simulink model "SetButton"  (R2017a)
settings: Solver=VariableStepAuto  StartTime=0.0  StopTime=60  RelTol=1e-3
libraries: arduino_io_lib x4, simulink x3, dspstat3 x1
settings Model: Creator=enes_  LastModifiedBy=enes_

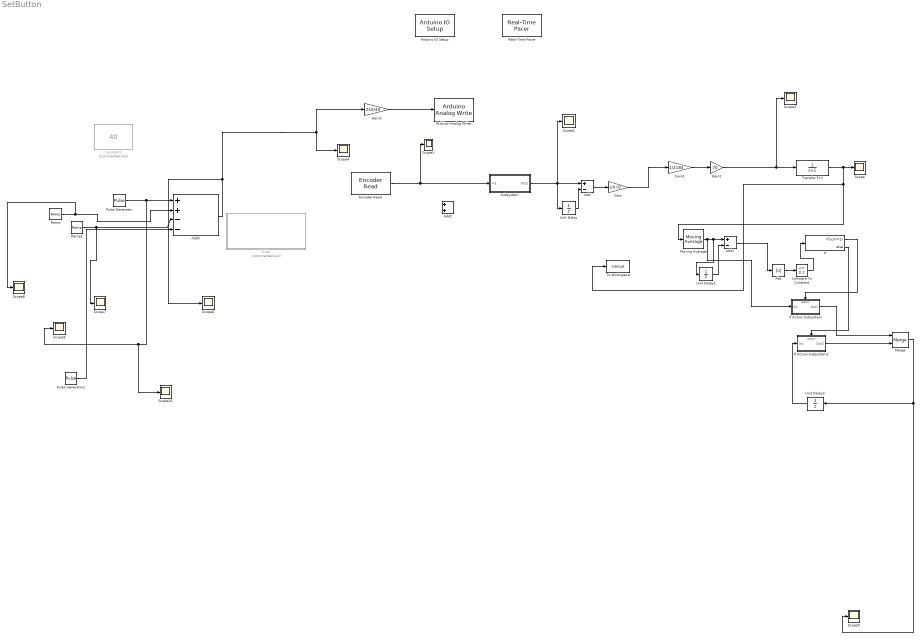
== system SetButton ==
  Abs : Abs
  Add : Sum  Inputs=+-
  Add1 : Sum  Inputs=+-
  Add2 : Sum
  Add3 : Sum  Inputs=++--
  Arduino Analog Write : arduino_io_lib/Arduino Analog Write  arduinoVar=Temporary arduino variable: Arduino1  arduinoPin=5  T=0.2
  Arduino IO Setup : arduino_io_lib/Arduino IO Setup  Priority=3  arduinoVar=Temporary arduino variable: Arduino1  workspaceVarName=a  comPort=COM4
  Compare To Constant : simulink/Logic and Bit Operations/Compare To Constant  relop=<=  const=0.2  OutDataTypeStr=boolean
  Constant1 : Constant  Commented=on  Value=40  SampleTime=0.02
  Encoder Read : arduino_io_lib/Encoder Read  arduinoVar=Temporary arduino variable: Arduino1  encNum=1  pinA=2  pinB=3  DbDl=1  T=0.02
  Gain : Gain  Gain=1/0.02
  Gain1 : Gain  Gain=1/2184
  Gain2 : Gain  Gain=70
  Gain3 : Gain  Gain=255/40
  If : If  IfExpression=u1==1
  If Action Subsystem : Subsystem  TreatAsAtomicUnit=on
  If Action Subsystem1 : Subsystem  TreatAsAtomicUnit=on
  Merge : Merge
  Moving Average : dspstat3/Moving Average  Method=Sliding window  SpecifyWindowLength=on  WindowLength=40  ForgettingFactor=0.9  SimulateUsing=Code generation
  Pulse Generator : DiscretePulseGenerator  Amplitude=0  Period=10  PulseWidth=10  PhaseDelay=40
  Pulse Generator1 : DiscretePulseGenerator  Amplitude=-40  Period=10  PulseWidth=10
  Ramp : simulink/Sources/Ramp  slope=1  start=0  X0=0
  Ramp1 : simulink/Sources/Ramp  slope=1  start=40  X0=40
  Real-Time Pacer : arduino_io_lib/Real-Time Pacer  simTimePerRealTime=1
  Scope{,1..10} (11 alike) : Scope
  Slider : Subsystem  Commented=on  DialogController=hmiCreateDDGDialog  IsWebBlock=on  mask(MWDashboardBlock){webBlockId=d8bc7804-6bab-4972-ab32-33c45766c117, webBlockType=slider, ShowInLibBrowser=on, ShowInitialText=on, HMISrcModelName=SetButton}
      mask prompts: webBlockId "WebBlock Id"; webBlockType "WebBlock Type"; HMISrcModelName "Source Model"
      mask help: SimulinkHMI:dialogs:SliderDialogDesc
      mask Help: helpview([docroot '/mapfiles/simulink.map'], 'hmi_slider')
      mask Display:
      | if strcmp(get_param(bdroot(gcb),'BlockDiagramType'), 'library')
      |     image([(matlabroot) '/toolbox/simulink/hmi/icons/Slider.png']);
      | end
  Subsystem : Subsystem
  To Workspace : ToWorkspace  VariableName=simout  SaveFormat=Timeseries  SampleTime=-1
  Transfer Fcn : TransferFcn  Denominator=[1 1]
  Unit Delay : UnitDelay  SampleTime=-1
  Unit Delay1 : UnitDelay  SampleTime=-1
  Unit Delay2 : UnitDelay  SampleTime=-1
  wires:
  Unit Delay/1 -> Add/2
  Add/1 -> Gain/1
  Gain/1 -> Gain1/1
  Gain1/1 -> Gain2/1
  Subsystem/1(Out1) -> Unit Delay/1, Scope2/1, Add/1
  Gain2/1 -> Transfer Fcn/1, Scope3/1
  Gain3/1 -> Arduino Analog Write/1
  Moving Average/1 -> If Action Subsystem/1(In1), Unit Delay1/1, Add1/1
  Unit Delay1/1 -> Add1/2
  Add1/1 -> Abs/1
  Abs/1 -> Compare To Constant/1
  Compare To Constant/1 -> If/1
  If/1 -> If Action Subsystem/Action
  If/2 -> If Action Subsystem1/Action
  If Action Subsystem/1(Out1) -> Merge/1
  Add3/1 -> Scope6/1, Scope4/1, Gain3/1
  If Action Subsystem1/1(Out1) -> Merge/2
  Merge/1 -> Unit Delay2/1, Scope5/1
  Transfer Fcn/1 -> To Workspace/1, Moving Average/1, Scope/1
  Encoder Read/1 -> Subsystem/1(In1), Scope1/1
  Pulse Generator/1 -> Scope10/1, Scope9/1, Add3/1
  Ramp/1 -> Scope8/1, Add3/2
  Ramp1/1 -> Scope7/1, Add3/3
  Pulse Generator1/1 -> Add3/4
  Unit Delay2/1 -> If Action Subsystem1/1(In1)

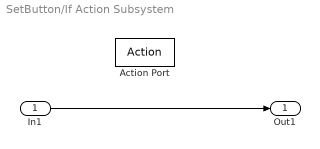
== system SetButton/If Action Subsystem ==
  In1 : Inport
  Action Port : ActionPort  ActionType=then
  Out1 : Outport
  wires:
  In1/1 -> Out1/1

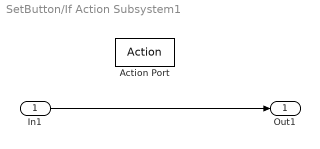
== system SetButton/If Action Subsystem1 ==
  In1 : Inport
  Action Port : ActionPort  ActionType=else
  Out1 : Outport
  wires:
  In1/1 -> Out1/1

== system SetButton/Slider ==

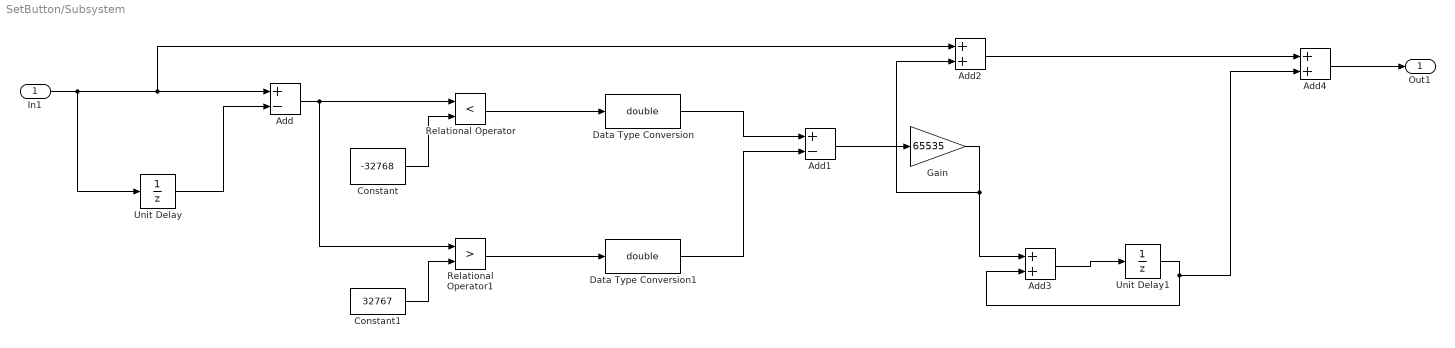
== system SetButton/Subsystem ==
  In1 : Inport
  Add : Sum  Inputs=+-
  Add1 : Sum  Inputs=+-
  Add2 : Sum
  Add3 : Sum
  Add4 : Sum
  Constant : Constant  Value=-32768
  Constant1 : Constant  Value=32767
  Data Type Conversion : DataTypeConversion  OutDataTypeStr=double
  Data Type Conversion1 : DataTypeConversion  OutDataTypeStr=double
  Gain : Gain  Gain=65535
  Relational Operator : RelationalOperator  Operator=<  OutDataTypeStr=boolean  RndMeth=Simplest
  Relational Operator1 : RelationalOperator  Operator=>  OutDataTypeStr=boolean  RndMeth=Simplest
  Unit Delay : UnitDelay  SampleTime=-1
  Unit Delay1 : UnitDelay  SampleTime=-1
  Out1 : Outport
  wires:
  In1/1 -> Add2/1, Add/1, Unit Delay/1
  Unit Delay/1 -> Add/2
  Constant/1 -> Relational Operator/2
  Add/1 -> Relational Operator1/1, Relational Operator/1
  Constant1/1 -> Relational Operator1/2
  Relational Operator1/1 -> Data Type Conversion1/1
  Relational Operator/1 -> Data Type Conversion/1
  Data Type Conversion/1 -> Add1/1
  Data Type Conversion1/1 -> Add1/2
  Add1/1 -> Gain/1
  Add2/1 -> Add4/1
  Gain/1 -> Add3/1, Add2/2
  Add4/1 -> Out1/1
  Add3/1 -> Unit Delay1/1
  Unit Delay1/1 -> Add4/2, Add3/2
